simulink model "xpcdspspectrum"  (Simulink 6.0)
settings: Solver=FixedStepDiscrete  SolverMode=MultiTasking  StartTime=0.0  StopTime=inf  RelTol=1e-3
libraries: dspbuff3 x2, dspsigattribs x2, dspsrcs4 x1, dspxfrm3 x1, simulink x1, xpclib x1, dspsigops x1
settings Model: Creator=mvetsch  LastModifiedBy=ekbas  ExtModeArmWhenConnect=off  BufferReuse=off
settings DataIOCC: SignalLoggingName=logsOut
settings OptimizationCC: BlockReduction=off  BooleanDataType=off  InlineInvariantSignals=off  OptimizeBlockIOStorage=off  BufferReuse=off  LocalBlockOutputs=off  ParameterPooling=off
settings DebuggingCC: CheckExecutionContextPreStartOutputMsg=on  CheckExecutionContextRuntimeOutputMsg=on  SolverPrmCheckMsg=none
settings RTWCC: SystemTargetFile=xpctarget.tlc  TemplateMakefile=xpc_default_tmf  ProcessScript=xpctarget_make_rtw_hook
settings xpcTargetCC: TargetFcnLib=ansi_tfl_tmw.mat  GenFloatMathFcnCalls=ANSI_C  ModelReferenceCompliant=off  LifeSpan=inf
settings SFSimCC: SFSimApplyToAllLibs=on  SFSimBuildMode=Incremental

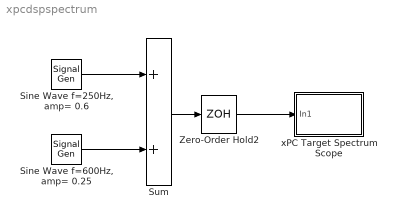
== system xpcdspspectrum ==
  "Sine Wave f=250Hz, amp= 0.6" : SignalGenerator  Amplitude=0.6  Frequency=200
  "Sine Wave f=600Hz, amp= 0.25" : SignalGenerator  Amplitude=0.25  Frequency=600
  Sum : Sum  SaturateOnIntegerOverflow=on  InputSameDT=on
  Zero-Order Hold2 : ZeroOrderHold  SampleTime=0.0005
  xPC Target Spectrum Scope : Subsystem  PropExecContextAcrossSSBoundary=on  mask(spectrum){N=512, scopetype=Target, axeslimits=[0,0.7]}
      mask prompts: N "Length of FFT:"; scopetype "Scope Type:"; axeslimits "Y-Axis Limits:"
      mask init:
      | N=2^(3+N);
      | if scopetype==1
      | set_param([gcb,'/Scope (xPC) '],'scopetype','Host');
      | elseif scopetype==2
      | set_param([gcb,'/Scope (xPC) '],'scopetype','Target');
      | end
      mask StyleString: popup(16|32|64|128|256|512|1024),popup(Host|Target),edit
      mask Display: disp('Spectrum')
  wires:
  Zero-Order Hold2/1 -> xPC Target Spectrum Scope/1(In1)
  Sum/1 -> Zero-Order Hold2/1
  "Sine Wave f=250Hz, amp= 0.6"/1 -> Sum/1
  "Sine Wave f=600Hz, amp= 0.25"/1 -> Sum/2

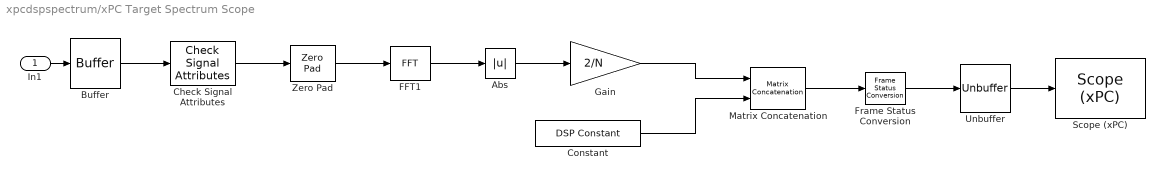
== system xpcdspspectrum/xPC Target Spectrum Scope ==
  In1 : Inport  LatchInput=off
  Abs : Abs  SaturateOnIntegerOverflow=on
  Buffer : dspbuff3/Buffer  N=N  V=0  ic=0
  Check Signal Attributes : dspsigattribs/Check Signal Attributes  SigAttribCheckMethod=Does not match attributes exactly  Complexity=Ignore  Frame=Frame-based  DimsCheckMethod=Is...  Dimensions=Column vector (2-D)  DatatypeCheckMethod=Ignore  DatatypeGeneral=Boolean  DtypeFloatSpecific=Any floating-point  DtypeFixedSpecific=Any fixed-point  DtypeIntSpecific=Any integer  SampleMode=Ignore
  Constant : dspsrcs4/DSP Constant  Value=[0.01;zeros(N-1,1)]  SampleMode=Discrete  discreteOutput=Sample-based  continuousOutput=Sample-based  sampTime=-1  framePeriod=-1  dataType=Inherit from 'Constant value'  isSigned=on  wordLen=16  udDataType=sfix(16)  fracBitsMode=Best precision  numFracBits=15  InterpretAs1D=off  Ts=-1  FramebasedOutput=off
  FFT1 : dspxfrm3/FFT  DialogController=dspDDGCreate  DialogControllerArgs=DataTag0  CompMethod=Table lookup  TableOpt=Speed  BitRevOrder=off  SkipNorm=on  roundingMode=Floor  overflowMode=off
  Frame Status Conversion : dspsigattribs/Frame Status Conversion  growRefPort=off  outframe=Frame-based
  Gain : Gain  Gain=2/N  SaturateOnIntegerOverflow=on
  Matrix Concatenation : simulink/Math Operations/Matrix Concatenation  numInports=2  catMethod=Horizontal
  "Scope (xPC) " : xpclib/Misc./Scope (xPC)   scopeno=1  scopetype=Target  autostart=on  viewmode=Graphical redraw  formatstr='%15.6f'  grid=on  ylimits=axeslimits  nosamples=N/2  noprepostsamples=0  interleave=1  triggermode=Signal triggering  triggersignal=2  triggerlevel=0.005  triggerslope=Rising  triggerscope=1  triggersample=0  filename=data.dat  mode=Lazy  writesize=512  autorestart=off
  Unbuffer : dspbuff3/Unbuffer  ic=0
  Zero Pad : dspsigops/Zero Pad  padSigAt=End  zpadAlong=Columns  padNumOutRowsSpecMethod=User-specified  numOutRows=N  padNumOutColsSpecMethod=User-specified  numOutCols=1  trunc_flag=None
  wires:
  Unbuffer/1 -> "Scope (xPC) "/1
  Constant/1 -> Matrix Concatenation/2
  Matrix Concatenation/1 -> Frame Status Conversion/1
  Frame Status Conversion/1 -> Unbuffer/1
  In1/1 -> Buffer/1
  Check Signal Attributes/1 -> Zero Pad/1
  Zero Pad/1 -> FFT1/1
  FFT1/1 -> Abs/1
  Buffer/1 -> Check Signal Attributes/1
  Abs/1 -> Gain/1
  Gain/1 -> Matrix Concatenation/1
